simulink model "modelPI"  (Simulink 8.9)
settings: Solver=ode45  StartTime=0.0  StopTime=25  MaxStep=1/60  RelTol=1e-6  EnableMultiTasking=on
values from neighbouring files (symbols this model uses):
  h = 1    [optymalizacja.m]    (also in optymalizacjaNastaw.m; parametry.m)
undefined symbols (not defined in the file or in its folder): sigbuilder_block
libraries: dsparch4 x1, simulink x1
settings Model: Creator=Krzys  LastModifiedBy=Szwank
settings DebuggingCC: SolverPrmCheckMsg=warning
settings GRTTargetCC: GeneratePreprocessorConditionals=Use local settings

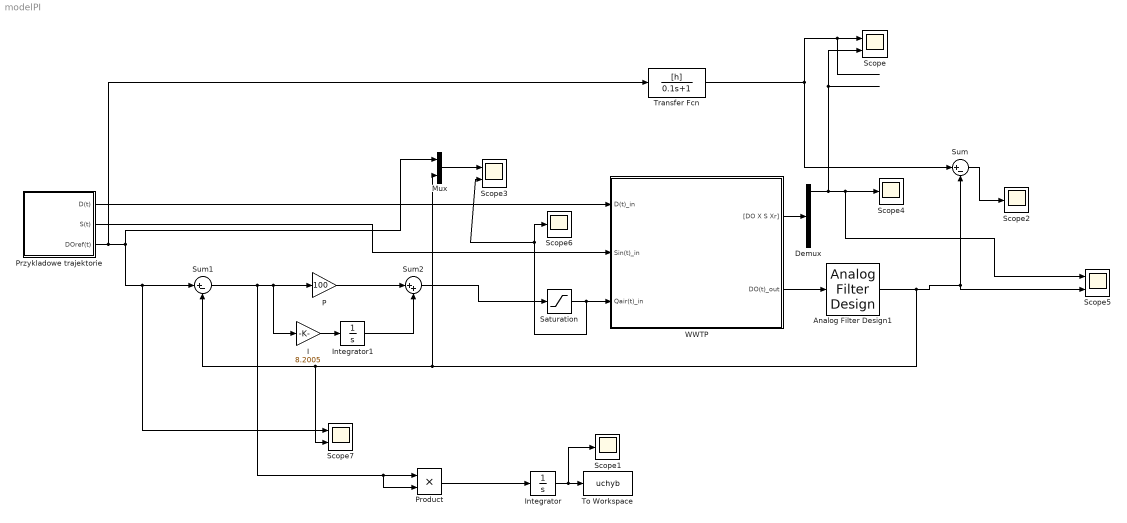
== system modelPI ==
  Analog Filter Design1 : dsparch4/Analog Filter Design  method=Chebyshev II  filttype=Lowpass  N=7  Wlo=90  Whi=80  Rp=10  Rs=50
  Demux : Demux
  I : Gain  Gain=8.2005
  Integrator : Integrator
  Integrator1 : Integrator
  Mux : Mux  Inputs=2
  P : Gain  Gain=100
  Product : Product
  Przykladowe trajektorie : Subsystem  Tag=STV Subsys  LoadFcn=sigbuilder_block('load');  StartFcn=sigbuilder_block('start');  StopFcn=sigbuilder_block('stop');  ClipboardFcn=sigbuilder_block('clipboard');  mask(Sigbuilder block){tuvar=[0:10]}
      mask help: Sigbuilder GUI
      mask init:
      | if ~strcmp(get_param(bdroot(gcbh),'SimulationStatus'),'stopped') tuvar = sigbuilder_block('maskInit'); end
      settings: CopyFcn=sigbuilder_block('copy');  DeleteFcn=sigbuilder_block('delete');  ModelCloseFcn=sigbuilder_block('modelClose');  PreSaveFcn=sigbuilder_block('preSave');  PauseFcn=sigbuilder_block('pause')  ContinueFcn=sigbuilder_block('continue')  NameChangeFcn=sigbuilder_block('namechange');  OpenFcn=sigbuilder_block('open',[377.25 224.25 550.5 399.75 ]);  CloseFcn=sigbuilder_block('close');
      mask Display: plot(0, 0, 100, 100,[2, 2, 32, 32, 2], [68, 8, 8, 68, 68],[32, 2], [38, 38], [32, 19, 2],[53, 60, 44], [32, 17, 17, 2],[16, 16, 31, 31]);txt = getActiveGroup(gcbh);text(2, 100, txt,'verticalAlignment', 'top');
  Saturation : Saturate  UpperLimit=300  LowerLimit=0
  Scope{,3,5,7} (4 alike) : Scope  NumInputPorts=2
  Scope{1..2,4,6} (4 alike) : Scope
  Sum : Sum  Inputs=|+-
  Sum1 : Sum  Inputs=|+-
  Sum2 : Sum  Inputs=|++
  To Workspace : ToWorkspace  VariableName=uchyb  SampleTime=-1
  Transfer Fcn : TransferFcn  Numerator=[h]  Denominator=[0.1 1]
  WWTP : Subsystem  mask{stateX=1225, stateS=20, stateDO=6, stateXr=2333}
  wires:
  Transfer Fcn/1 -> Sum/1, Scope/1
  Przykladowe trajektorie/3(DOref(t)) -> Transfer Fcn/1, Scope7/1, Sum1/1, Mux/1
  WWTP/1("[DO X S Xr]") -> Demux/1
  Przykladowe trajektorie/1(D(t)) -> WWTP/1(D(t)_in)
  Przykladowe trajektorie/2(S(t)) -> WWTP/2(Sin(t)_in)
  Sum/1 -> Scope2/1
  Mux/1 -> Scope3/1
  Analog Filter Design1/1 -> Mux/2, Scope7/2, Sum1/2, Sum/2, Scope5/2
  WWTP/2(DO(t)_out) -> Analog Filter Design1/1
  P/1 -> Sum2/1
  Demux/1 -> Scope/2, Scope5/1, Scope4/1
  Product/1 -> Integrator/1
  Integrator/1 -> Scope1/1, To Workspace/1
  Sum1/1 -> Product/2, Product/1, I/1, P/1
  I/1 -> Integrator1/1
  Integrator1/1 -> Sum2/2
  Saturation/1 -> Scope3/2, Scope6/1, WWTP/3(Qair(t)_in)
  Sum2/1 -> Saturation/1

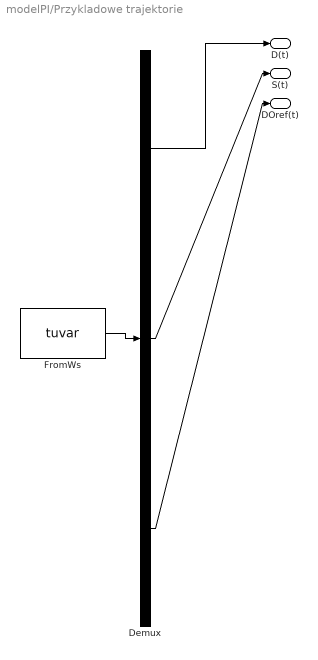
== system modelPI/Przykladowe trajektorie ==
  Demux : Demux  Tag=STV Demux  Outputs=3
  FromWs : FromWorkspace  Tag=STV FromWs  VariableName=tuvar  SampleTime=0  SigBuilderData=DataTag0  VnvData=DataTag1
      SigBuilderData=|
      | common.afterFinalStr = 'Extrapolate'
      | common.sampleTime = 0
      | dataSet.timeRange = [0 24]
      | dataSet.name = 'Group 1'
      | sbobj.Groups.Name = 'Group 1'
      | sbobj.Groups.Signals(1).Name = 'D(t)'
      | sbobj.Groups.Signals(1).XData = [0 4 4 7 7 12 12 16 16 20 20 24]
      | sbobj.Groups.Signals(1).YData = [0.065 0.065 0.025 0.025 0.05 0.05 0.04 0.04 0.065 0.065 0.03 0.03]
      | sbobj.Groups.Signals(2).Name = 'S(t)'
      | sbobj.Groups.Signals(2).XData = [0 4 4 7 7 12 12 16 16 20 20 24]
      | sbobj.Groups.Signals(2).YData = [600 600 200 200 500 500 400 400 600 600 350 350]
      | sbobj.Groups.Signals(3).Name = 'DOref(t)'
      | sbobj.Groups.Signals(3).XData = [0 2 2 4 4 6 6 8 8 10 10 12 12 14 14 16 16 18 18 20 20 22 22 24]
      | sbobj.Groups.Signals(3).YData = [1.5 1.5 9.4 9.4 5 5 2 2 2.5 2.5 7 7 2.5 2.5 4 4 8.5 8.5 6 6 2 2 3 3]
      | sbobj.Groups.TimeRange = [0 24]
  D(t) : Outport  Tag=STV Outport
  S(t) : Outport  Tag=STV Outport  Port=2
  DOref(t) : Outport  Tag=STV Outport  Port=3
  wires:
  Demux/1 -> D(t)/1
  FromWs/1 -> Demux/1
  Demux/2 -> S(t)/1
  Demux/3 -> DOref(t)/1

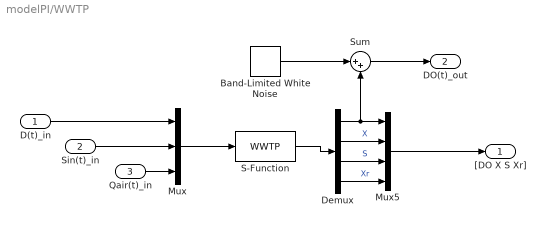
== system modelPI/WWTP ==
  D(t)_in : Inport
  Sin(t)_in : Inport  Port=2
  Qair(t)_in : Inport  Port=3
  Band-Limited White Noise : simulink/Sources/Band-Limited White Noise  Cov=[0.001]  Ts=1/60  seed=[23341]
  Demux : Demux
  Mux : Mux  Inputs=3
  Mux5 : Mux
  S-Function : S-Function  FunctionName=WWTP  Parameters=stateX stateS stateDO stateXr  SFunctionDeploymentMode=off  EnableBusSupport=off
  Sum : Sum  Inputs=|++
  "[DO X S Xr]" : Outport
  DO(t)_out : Outport  Port=2
  wires:
  D(t)_in/1 -> Mux/1
  Sin(t)_in/1 -> Mux/2
  Qair(t)_in/1 -> Mux/3
  Mux/1 -> S-Function/1
  S-Function/1 -> Demux/1
  Demux/2 -> Mux5/2  "X"
  Demux/3 -> Mux5/3  "S"
  Demux/4 -> Mux5/4  "Xr"
  Demux/1 -> Mux5/1, Sum/2
  Band-Limited White Noise/1 -> Sum/1
  Sum/1 -> DO(t)_out/1
  Mux5/1 -> "[DO X S Xr]"/1
